simulink model "controller"  (R2021a)
settings: Solver=FixedStepAuto  StartTime=0.0  StopTime=25  FixedStep=0.1  RelTol=1e-3  EnableMultiTasking=on
values from neighbouring files (symbols this model uses):
  theta = -45    [car.m]
libraries: fuzblock x1
settings Model: Creator=Gregory  LastModifiedBy=Administrator
settings SolverCC: AlgebraicLoopSolver=TrustRegion
settings DataIOCC: SaveFormat=Array  ReturnWorkspaceOutputs=off  OutputOption=SpecifiedOutputTimes  OutputTimes=[0.01:0.01:10]
settings OptimizationCC: LifeSpan=inf
settings DebuggingCC: UnderspecifiedInitializationDetection=Classic  MergeDetectMultiDrivingBlocksExec=none  SolverPrmCheckMsg=warning  StateNameClashWarn=warning  SFUnexpectedBacktrackingDiag=warning  SFNoUnconditionalDefaultTransitionDiag=warning  SFMachineParentedDataDiag=warning  ArithmeticOperatorsInVariantConditions=warning
settings HardwareCC: ProdBitPerPointer=32  ProdBitPerSizeT=32  ProdBitPerPtrDiffT=32  ProdLargestAtomicFloat=None  ProdIntDivRoundTo=Undefined  ProdEndianess=Unspecified  ProdWordSize=32  ProdHWDeviceType=32-bit Generic
settings ModelReferenceCC: PropagateSignalLabelsOutOfModel=off
settings SFSimCC: SimUseLocalCustomCode=off  CustomCodeUndefinedFunction=UseInterfaceOnly
settings RTWCC: RTWUseLocalCustomCode=off
settings CodeAppCC: StateflowObjectComments=on
settings GRTTargetCC: TargetLangStandard=C89/C90 (ANSI)
settings ConfigComp: CovMetricSettings=dw  CovSaveCumulativeToWorkspaceVar=on  CovSaveSingleToWorkspaceVar=on  CovExternalEMLEnable=off

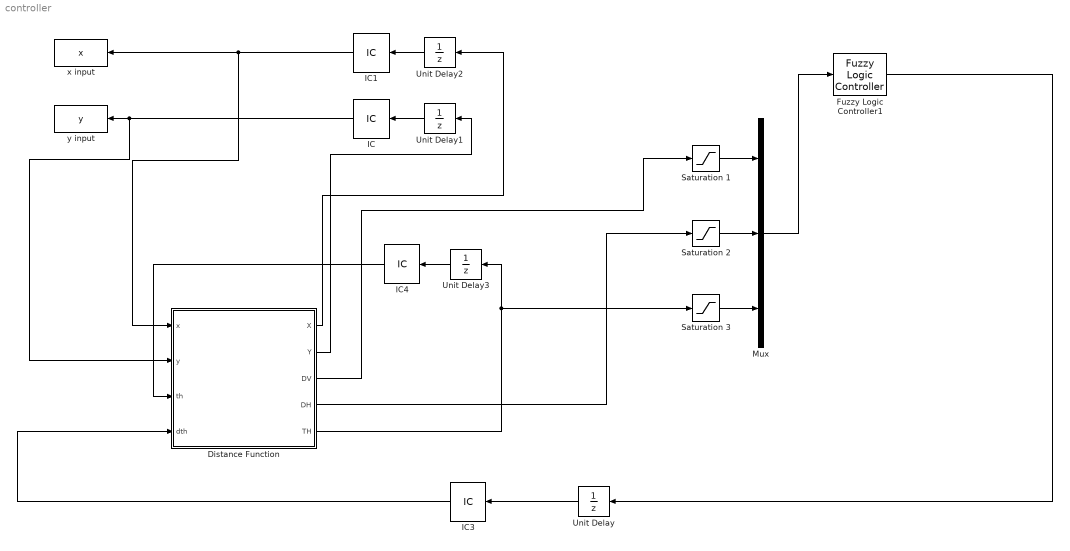
== system controller ==
  Distance Function : MATLAB Function  TreatAsAtomicUnit=on
  Fuzzy Logic Controller1 : fuzblock/Fuzzy Logic  Controller  FIS='FLC2.fis'  OutputSampleNumber=101  DataType=double  FuzzifiedInputs=off  RuleFiringStrengths=off  RuleOutputs=off  AggregatedOutputs=off  SimulateUsing=Interpreted execution  OutOfRangeInputValueMessage=warning  NoRuleFiredMessage=warning  EmptyOutputFuzzySetMessage=warning
  IC : InitialCondition  Value=0.4
  IC1 : InitialCondition  Value=4
  IC3 : InitialCondition  Value=0
  IC4 : InitialCondition  Value=theta
  Mux : Mux  Inputs=3
  Saturation 1 : Saturate  UpperLimit=1  LowerLimit=0
  Saturation 2 : Saturate  UpperLimit=1  LowerLimit=0
  Saturation 3 : Saturate  UpperLimit=180  LowerLimit=-180
  Unit Delay{,1..3} (4 alike) : UnitDelay  SampleTime=-1  HasFrameUpgradeWarning=on
  x input : ToWorkspace  VariableName=x  SampleTime=-1
  y input : ToWorkspace  VariableName=y  SampleTime=-1
  wires:
  Distance Function/1(X) -> Unit Delay2/1
  Distance Function/2(Y) -> Unit Delay1/1
  IC/1 -> Distance Function/2(y), y input/1
  IC1/1 -> x input/1, Distance Function/1(x)
  IC3/1 -> Distance Function/4(dth)
  Mux/1 -> Fuzzy Logic Controller1/1
  Fuzzy Logic Controller1/1 -> Unit Delay/1
  Unit Delay/1 -> IC3/1
  Unit Delay1/1 -> IC/1
  Unit Delay2/1 -> IC1/1
  Distance Function/3(DV) -> Saturation 1/1
  Distance Function/4(DH) -> Saturation 2/1
  Saturation 1/1 -> Mux/1
  Saturation 2/1 -> Mux/2
  Saturation 3/1 -> Mux/3
  Unit Delay3/1 -> IC4/1
  IC4/1 -> Distance Function/3(th)
  Distance Function/5(TH) -> Unit Delay3/1, Saturation 3/1

== matlab function controller/Distance Function ==
  data: x input; y input; th input; X output; Y output; DV output; DH output; TH output; dth input
function [X, Y, DV, DH, TH] = fcn(x, y, th, dth)

TH= th + dth;

if TH > 180
    TH = -360 + TH;
elseif TH < -180
    TH = 360 + TH;
end

if x < 10
    X = x + 0.05*cosd(TH);
    Y = y + 0.05*sind(TH);
else
    X = x;
    Y = y;
end;

[DH, DV] = f(X, Y);
end


function [dH, dV]= f(x,y)
    if (x < 5)
        dV = y;
    elseif (x < 6)
        dV = y - 1;
    elseif (x < 7)
        dV = y - 2;
    else
        dV = y - 3;
    end

    
    if (y < 1)
        dH = 5 - x;
    elseif (y < 2)
        dH = 6 - x;
    elseif (y < 3)
        dH = 7 - x;
    else
        dH = 10;
    end
end
